simulink model "ReactionWheel_Sim_1"  (R2024b)
settings: Solver=VariableStepAuto  StartTime=0.0  StopTime=10.0  RelTol=1e-3
values from neighbouring files (symbols this model uses):
  b = 0.000178    [Controller.m]    (also in FeetForward_Controller.mat; ReactionWheelModel1.m; run_FIRST.m = 3.97e-06)
  DCM_BODY_wrt_RW = [ 0.408248 0.408248 -0.816496 ... (first row only)    [Controller.m]    (also in FeetForward_Controller.mat = [0.408248  0.408248  -0.816496; -0.7071  0.7071  0; 0.5774  ; ReactionWheelModel1.m)
  dtrw = 0.05    [Controller.m]    (also in FeetForward_Controller.mat; ReactionWheelModel1.m)
  I_rw = [I_a 0 0; 0 I_a 0; 0 0 I_a]    [Controller.m]    (also in FeetForward_Controller.mat = [0.0725  0  0; 0  0.0725  0; 0  0  0.0725]; ReactionWheelModel1.m)
  Iab = [Ixx 0 0 ... (first row only)    [Controller.m]    (also in FeetForward_Controller.mat = [4.0774  0  0; 0  4.136  0; 0  0  2.3216]; ReactionWheelModel1.m)
  J = 0.00725    [Controller.m]    (also in FeetForward_Controller.mat; ReactionWheelModel1.m; run_FIRST.m = 0.0001)
  K_e = 0.071    [Controller.m]    (also in FeetForward_Controller.mat; ReactionWheelModel1.m)
  K_t = 0.070    (= 0.07)    [Controller.m]    (also in FeetForward_Controller.mat; ReactionWheelModel1.m; satellitemodel2711.m = 0.1)
  L = 0.00339    [Controller.m]    (also in FeetForward_Controller.mat; Model_2811.m = 0.001; ReactionWheelModel1.m; run_FIRST.m = 0.003)
  R = 1.52    [Controller.m]    (also in FeetForward_Controller.mat; Model_2811.m = 1; ReactionWheelModel1.m; run_FIRST.m = 0.141)
libraries: aerolibutil x1
settings Model: Creator=LEGION  LastModifiedBy=LEGION

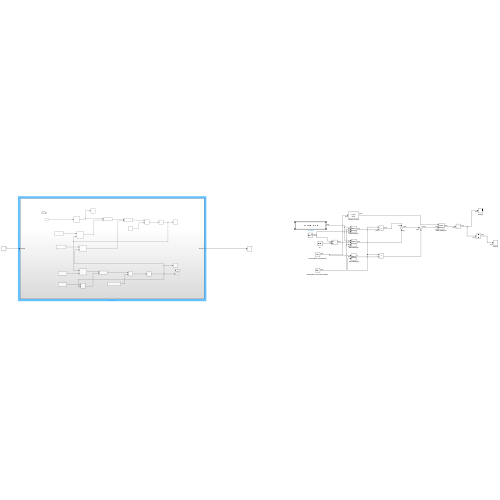
[thumbnail: Simulink's stored preview of the top-level diagram]
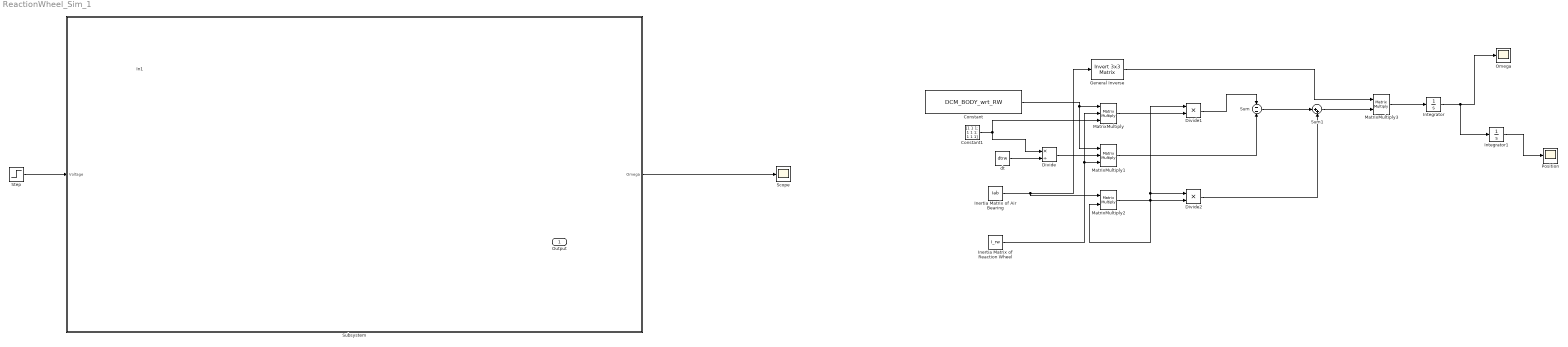
== system ReactionWheel_Sim_1 ==
  In1 : Inport
  Constant : Constant  Value=DCM_BODY_wrt_RW
  Constant1 : Constant  Value=[1 1 1; 1 1 1; 1 1 1]
  Divide : Product  Inputs=*/
  Divide1 : Product  Inputs=**
  Divide2 : Product  Inputs=**
  General Inverse : aerolibutil/Invert  3x3 Matrix
  "Inertia Matrix of Air Bearing " : Constant  Value=Iab
  "Inertia Matrix of Reaction Wheel " : Constant  Value=I_rw
  Integrator : Integrator
  Integrator1 : Integrator
  MatrixMultiply : Product  Inputs=3  Multiplication=Matrix(*)
  MatrixMultiply1 : Product  Inputs=3  Multiplication=Matrix(*)
  MatrixMultiply2 : Product  Multiplication=Matrix(*)
  MatrixMultiply3 : Product  Multiplication=Matrix(*)
  "Omega " : Scope
  Position : Scope
  Scope : Scope
  Step : Step  After=10  SampleTime=0
  Subsystem : Subsystem
  Sum : Sum  Inputs=--
  Sum1 : Sum  Inputs=|++
  dt : Constant  Value=dtrw
  Output : Outport
  wires:
  Step/1 -> Subsystem/1(Voltage)
  Subsystem/1(Omega) -> Scope/1
  dt/1 -> Divide/2
  Constant1/1 -> MatrixMultiply/3, Divide/1
  Constant/1 -> MatrixMultiply/1, MatrixMultiply1/1
  "Inertia Matrix of Reaction Wheel "/1 -> MatrixMultiply1/3, MatrixMultiply/2
  Divide/1 -> MatrixMultiply1/2
  "Inertia Matrix of Air Bearing "/1 -> MatrixMultiply2/1, General Inverse/1
  MatrixMultiply/1 -> Divide1/2
  Divide1/1 -> Sum/1
  MatrixMultiply1/1 -> Sum/2
  Sum/1 -> Sum1/1
  Divide2/1 -> Sum1/2
  Sum1/1 -> MatrixMultiply3/2
  General Inverse/1 -> MatrixMultiply3/1
  MatrixMultiply2/1 -> Divide2/1, Divide1/1, MatrixMultiply2/2, Divide2/2
  MatrixMultiply3/1 -> Integrator/1
  Integrator1/1 -> Position/1
  Integrator/1 -> Integrator1/1, "Omega "/1

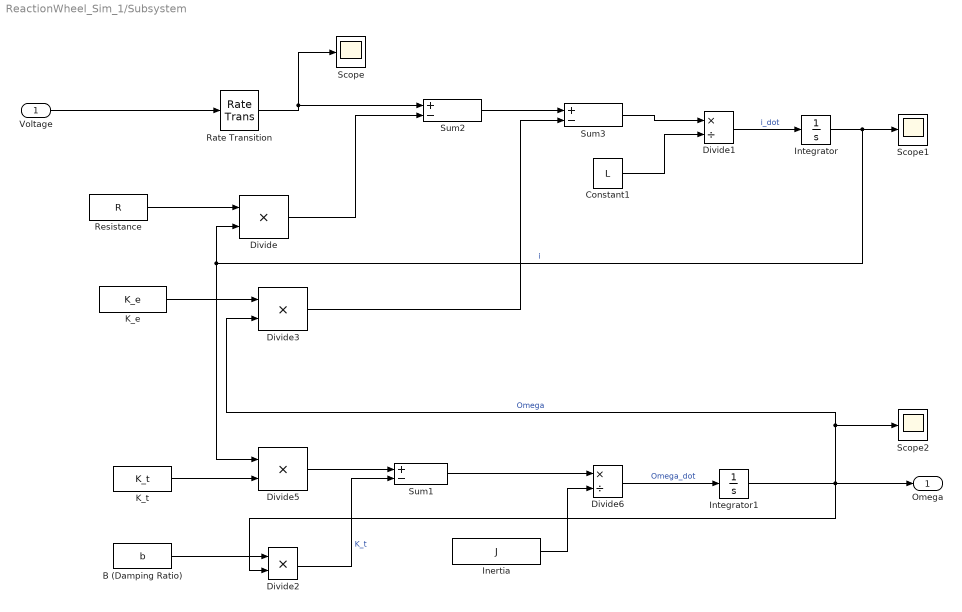
== system ReactionWheel_Sim_1/Subsystem ==
  Voltage : Inport
  B (Damping Ratio) : Constant  Value=b
  Constant1 : Constant  Value=L
  Divide{,2..3,5} (4 alike) : Product  Inputs=**
  Divide1 : Product  Inputs=*/
  Divide6 : Product  Inputs=*/
  Inertia : Constant  Value=J
  Integrator : Integrator
  Integrator1 : Integrator
  K_e : Constant  Value=K_e
  K_t : Constant  Value=K_t
  Rate Transition : RateTransition
  Resistance : Constant  Value=R
  Scope : Scope
  Scope1 : Scope
  Scope2 : Scope
  Sum1 : Sum  Inputs=+-
  Sum2 : Sum  Inputs=+-
  Sum3 : Sum  Inputs=+-
  Omega : Outport
  wires:
  Divide3/1 -> Sum3/2
  Divide2/1 -> Sum1/2  "K_t"
  Rate Transition/1 -> Scope/1, Sum2/1
  Sum2/1 -> Sum3/1
  Integrator/1 -> Divide5/1, Divide/2, Scope1/1  "i"
  K_t/1 -> Divide5/2
  Divide5/1 -> Sum1/1
  Divide/1 -> Sum2/2
  Resistance/1 -> Divide/1
  K_e/1 -> Divide3/1
  Divide1/1 -> Integrator/1  "i_dot"
  Divide6/1 -> Integrator1/1  "Omega_dot"
  Integrator1/1 -> Omega/1, Divide3/2, Scope2/1, Divide2/2  "Omega"
  Voltage/1 -> Rate Transition/1
  Constant1/1 -> Divide1/2
  Sum3/1 -> Divide1/1
  B (Damping Ratio)/1 -> Divide2/1
  Sum1/1 -> Divide6/1
  Inertia/1 -> Divide6/2
